simulink model "CrabRegulator"  (R2015a)
settings: Solver=ode23s  StartTime=0.0  StopTime=50  RelTol=1e-6  AbsTol=1e-9
settings Model: Creator=Utilisateur-pc  LastModifiedBy=ironi
settings DataIOCC: SignalLoggingSaveFormat=ModelDataLogs
settings OptimizationCC: ExpressionDepthLimit=2147483647
settings DebuggingCC: UnderspecifiedInitializationDetection=Classic  MergeDetectMultiDrivingBlocksExec=none  SolverPrmCheckMsg=warning  FcnCallInpInsideContextMsg=EnableAllAsWarning  StateNameClashWarn=warning
settings GRTTargetCC: CombineOutputUpdateFcns=off  GRTInterface=on

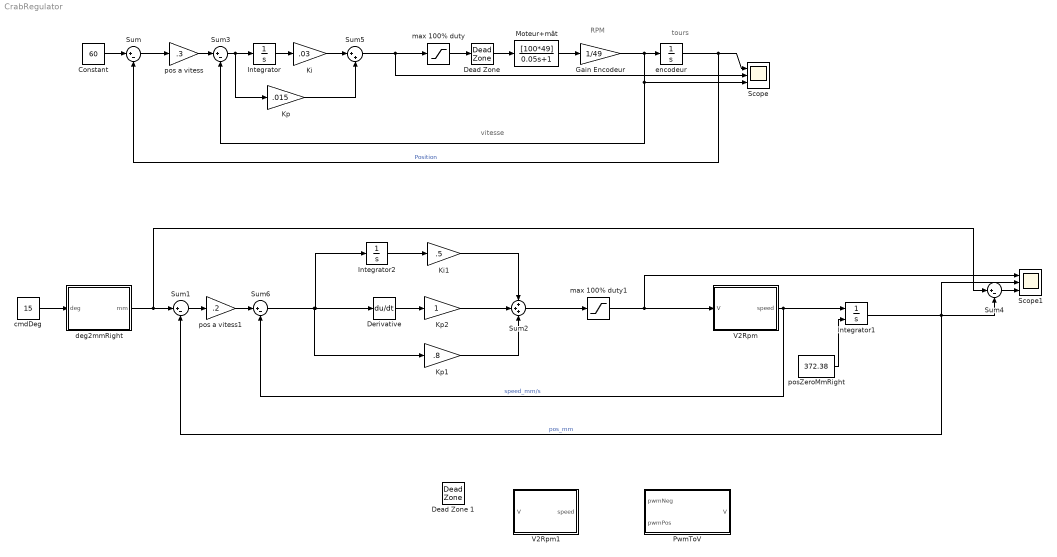
== system CrabRegulator ==
  note: RPM
  note: tours
  note: vitesse
  Constant : Constant  Value=60
  "Dead Zone " : DeadZone  LowerValue=-0.1  UpperValue=0.1  SaturateOnIntegerOverflow=on
  Dead Zone 1 : DeadZone  LowerValue=-0.1  UpperValue=0.1  SaturateOnIntegerOverflow=on
  Derivative : Derivative
  Gain Encodeur : Gain  Gain=1/49
  Integrator : Integrator
  Integrator1 : Integrator  InitialConditionSource=external
  Integrator2 : Integrator
  Ki : Gain  Gain=.03
  Ki1 : Gain  Gain=.5
  Kp : Gain  Gain=.015
  Kp1 : Gain  Gain=.8
  Kp2 : Gain
  Moteur+mât : TransferFcn  Numerator=[100*49]  Denominator=[0.05 1]
  PwmToV : MATLAB Function  TreatAsAtomicUnit=on
  Scope : Scope  NumInputPorts=3
      settings: YMin=-5~-5~-5  YMax=5~5~5
  Scope1 : Scope  NumInputPorts=3
      settings: YMin=-5~-5~-5  YMax=5~5~5
  Sum : Sum  Inputs=|+-  SampleTime=0.1
  Sum1 : Sum  Inputs=|+-  SampleTime=0.1
  Sum2 : Sum  Inputs=+++
  Sum3 : Sum  Inputs=|+-
  Sum4 : Sum  Inputs=|+-  SampleTime=0.1
  Sum5 : Sum  Inputs=|++
  Sum6 : Sum  Inputs=|+-
  V2Rpm : MATLAB Function  TreatAsAtomicUnit=on
  V2Rpm1 : MATLAB Function  TreatAsAtomicUnit=on
  cmdDeg : Constant  Value=15
  deg2mmRight : MATLAB Function  TreatAsAtomicUnit=on
  encodeur : Integrator
  max 100% duty : Saturate  UpperLimit=1  LowerLimit=-1
  max 100% duty1 : Saturate  UpperLimit=12  LowerLimit=-12
  pos a vitess : Gain  Gain=.3
  pos a vitess1 : Gain  Gain=.2
  posZeroMmRight : Constant  Value=372.38
  wires:
  V2Rpm/1(speed) -> Integrator1/1, Sum6/2  "speed_mm/s"
  posZeroMmRight/1 -> Integrator1/2
  cmdDeg/1 -> deg2mmRight/1(deg)
  Integrator1/1 -> Sum4/2, Sum1/2, Scope1/2  "pos_mm"
  Integrator2/1 -> Ki1/1
  Sum2/1 -> max 100% duty1/1
  max 100% duty1/1 -> Scope1/1, V2Rpm/1(V)
  deg2mmRight/1(mm) -> Sum4/1, Sum1/1
  Derivative/1 -> Kp2/1
  Ki1/1 -> Sum2/1
  Kp2/1 -> Sum2/2
  Kp1/1 -> Sum2/3
  Sum4/1 -> Scope1/3
  Moteur+mât/1 -> Gain Encodeur/1
  encodeur/1 -> Scope/1, Sum/2  "Position"
  Constant/1 -> Sum/1
  max 100% duty/1 -> "Dead Zone "/1
  "Dead Zone "/1 -> Moteur+mât/1
  pos a vitess/1 -> Sum3/1
  Sum3/1 -> Integrator/1, Kp/1
  Gain Encodeur/1 -> Scope/3, Sum3/2, encodeur/1
  Integrator/1 -> Ki/1
  Sum5/1 -> max 100% duty/1, Scope/2
  Kp/1 -> Sum5/2
  Sum/1 -> pos a vitess/1
  Ki/1 -> Sum5/1
  Sum1/1 -> pos a vitess1/1
  pos a vitess1/1 -> Sum6/1
  Sum6/1 -> Kp1/1, Integrator2/1, Derivative/1

== matlab function CrabRegulator/V2Rpm ==
  data: V input; speed output
function speed = fcn(V)

maxSpeed = 7.62;  % mm/s
maxVolt  = 12;  % V

speed = V/maxVolt * maxSpeed;

== matlab function CrabRegulator/PwmToV ==
  data: pwmNeg input; V output; pwmPos input
function V = fcn(pwmNeg, pwmPos)

V = 24*pwmPos + -24*pwmNeg;

== matlab function CrabRegulator/deg2mmRight ==
  data: deg input; mm output
function mm = fcn(deg)

% deg = round(deg, 0);
% 
% deg2mmRelRight = [53.68, 52.47, 51.25, 50, 48.74, 47.46, 46.16, 44.85, 43.51, 42.16, 40.79, 39.4, 37.99, 36.57, 35.12, 33.65, 32.16, 30.66, 29.13, 27.81, 26.02, 24.43, 22.82, 21.19, 19.54, 17.87, 16.18, 14.47, 12.74, 10.98, 9.2, 7.41, 5.59, 3.75, 1.89, 0, -1.9, -3.83, -5.77, -7.74, -9.73, -11.74, -13.77, -15.82, -17.89, -19.98, -22.09, -24.22, -26.36, -28.53, -30.72, -32.92, -35.14, -37.38, -39.63, -41.9, -44.19, -46.49, -48.81, -51.14, -53.48, -55.84, -58.21, -60.59, -62.98, -65.38, -67.79, -70.21, -72.63, -75.06, -77.5];
% posZeroMmRight = 372.38;
% deg2mmRight    = deg2mmRelRight + posZeroMmRight;
% 
% degList = -35:1:35;
% 
% % mmIndex = degList == deg;
% mmIndex = find(degList == deg);
% 
% mm = deg2mmRight(mmIndex);

mm = 341.66;

== matlab function CrabRegulator/V2Rpm1 ==
  data: V input; speed output
function speed = fcn(V)

maxSpeed = 7.62;  % mm/s
maxVolt  = 12;  % V

speed = V/maxVolt * maxSpeed;
